simulink subsystem "PieroControladorPosicion"  (R2023b)
settings: Solver=VariableStepAuto  StartTime=0.0  StopTime=10.0  RelTol=1e-3
undefined symbols (not defined in the file): DiscIntNeverNeededParam
settings Model: Creator=jaime  LastModifiedBy=jaime

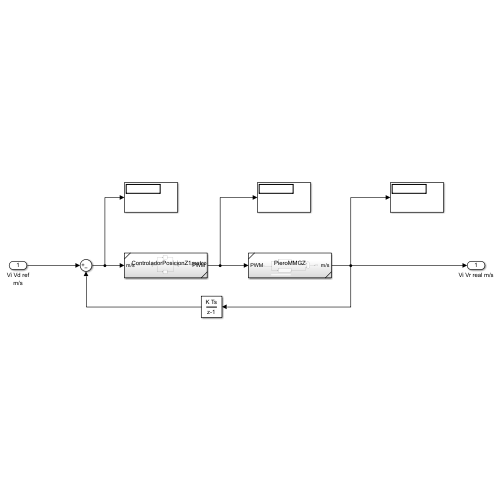
[thumbnail: Simulink's stored preview of the top-level diagram]
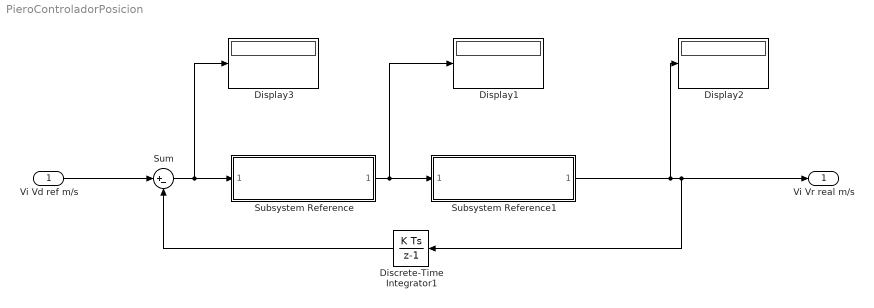
== system PieroControladorPosicion ==
  Vi Vd ref m/s : Inport  OutDataTypeStr=double  PortDimensions=2
  Discrete-Time Integrator1 : DiscreteIntegrator  SampleTime=-1  ICPrevOutput=DiscIntNeverNeededParam  ICPrevScaledInput=DiscIntNeverNeededParam
  Display1 : Display
  Display2 : Display
  Display3 : Display
  Subsystem Reference : Subsystem  ReferencedSubsystem=ControladorPosicionZ1metro
  Subsystem Reference1 : Subsystem  ReferencedSubsystem=PieroMMGZ
  Sum : Sum  Inputs=|+-
  Vi Vr real m/s : Outport  OutDataTypeStr=double  PortDimensions=2
  wires:
  Discrete-Time Integrator1/1 -> Sum/2
  Vi Vd ref m/s/1 -> Sum/1
  Subsystem Reference/1 -> Display1/1, Subsystem Reference1/1
  Sum/1 -> Subsystem Reference/1, Display3/1
  Subsystem Reference1/1 -> Display2/1, Vi Vr real m/s/1, Discrete-Time Integrator1/1
